simulink model "task4"  (R2021a)
settings: Solver=VariableStepAuto  StartTime=0.0  StopTime=10.0  RelTol=1e-3
settings Model: Creator=NoteBook  LastModifiedBy=NoteBook

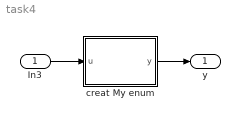
== system task4 ==
  In3 : Inport  OutDataTypeStr=Enum: enum1
  creat My enum : MATLAB Function  TreatAsAtomicUnit=on
  y : Outport
  wires:
  creat My enum/1(y) -> y/1
  In3/1 -> creat My enum/1(u)

== matlab function task4/creat My enum ==
  data: u input; y output
function y = fcn(u)
classdef enum1 < Simulink.IntEnumType
    enumeration
        ele1(1),
        ele2(2),
    end
end
y = u;
